simulink model "UkladNieZeroweWarunkiObaDyskretne"  (R2016a)
settings: Solver=ode45  StartTime=0.0  StopTime=10.0  MinStep=0.001  RelTol=1e-5
values from neighbouring files (symbols this model uses):
  GDyskretne = acker(systemDyskretny.A',systemDyskretny.C',[exp(T*-14),exp(T*-28),exp(T*-36)])'    [zad1.m]
  systemDyskretny = c2d(system,T,'foh')    [zad1.m]
settings Model: Creator=student  LastModifiedBy=student

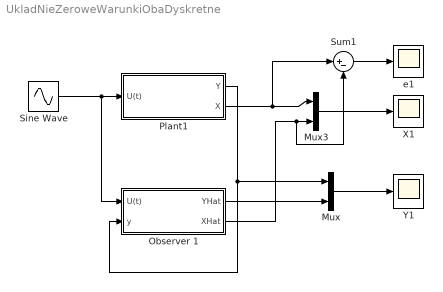
== system UkladNieZeroweWarunkiObaDyskretne ==
  Mux : Mux  Inputs=2
  Mux3 : Mux  Inputs=2
  Observer 1 : Subsystem
  Plant1 : Subsystem
  Sine Wave : Sin  SampleTime=0
  Sum1 : Sum  Inputs=|+-
  X1 : Scope
  Y1 : Scope
  e1 : Scope
  wires:
  Sine Wave/1 -> Observer 1/1(U(t)), Plant1/1(U(t))
  Plant1/1(Y) -> Mux/1, Observer 1/2("y ")
  Plant1/2(X) -> Sum1/1, Mux3/1
  Observer 1/2(XHat) -> Sum1/2, Mux3/2
  Mux3/1 -> X1/1
  Mux/1 -> Y1/1
  Sum1/1 -> e1/1
  Observer 1/1(YHat) -> Mux/2

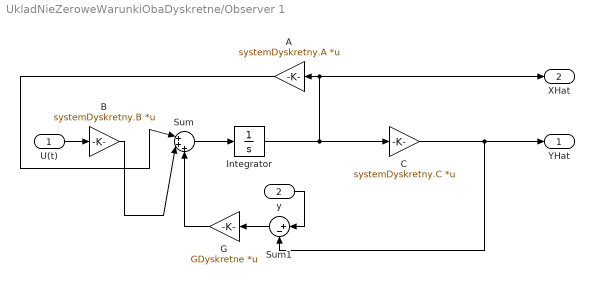
== system UkladNieZeroweWarunkiObaDyskretne/Observer 1 ==
  U(t) : Inport
  "y " : Inport  Port=2
  A : Gain  Gain=systemDyskretny.A  Multiplication=Matrix(K*u)
  B : Gain  Gain=systemDyskretny.B  Multiplication=Matrix(K*u)
  C : Gain  Gain=systemDyskretny.C  Multiplication=Matrix(K*u)
  G : Gain  Gain=GDyskretne  Multiplication=Matrix(K*u)
  Integrator : Integrator  InitialCondition=[1 1 1]
  Sum : Sum  Inputs=|+++
  Sum1 : Sum  Inputs=|+-
  YHat : Outport
  XHat : Outport  Port=2
  wires:
  A/1 -> Sum/1
  U(t)/1 -> B/1
  Integrator/1 -> C/1, XHat/1, A/1
  C/1 -> Sum1/2, YHat/1
  B/1 -> Sum/2
  Sum/1 -> Integrator/1
  "y "/1 -> Sum1/1
  Sum1/1 -> G/1
  G/1 -> Sum/3

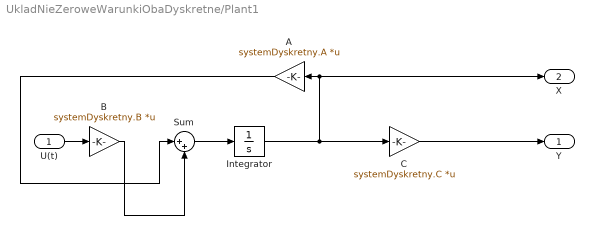
== system UkladNieZeroweWarunkiObaDyskretne/Plant1 ==
  U(t) : Inport
  A : Gain  Gain=systemDyskretny.A  Multiplication=Matrix(K*u)
  B : Gain  Gain=systemDyskretny.B  Multiplication=Matrix(K*u)
  C : Gain  Gain=systemDyskretny.C  Multiplication=Matrix(K*u)
  Integrator : Integrator
  Sum : Sum  Inputs=|++
  Y : Outport
  X : Outport  Port=2
  wires:
  A/1 -> Sum/1
  U(t)/1 -> B/1
  Integrator/1 -> C/1, X/1, A/1
  C/1 -> Y/1
  B/1 -> Sum/2
  Sum/1 -> Integrator/1
